simulink model "twoaxis_camera_gantry_Solution_OHackett"  (R2021b)
settings: Solver=ode23t  StartTime=0.0  StopTime=50  MaxStep=0.01  RelTol=1e-3  EnableMultiTasking=on
model workspace: external: MATLAB File gantryParams.m (data not in the file)
values from neighbouring files (symbols this model uses):
  endSupport = struct    [gantryParams.m]
  endSupportZ = struct    [gantryParams.m]
  leadScrew = struct    [gantryParams.m]
  leadScrewZ = struct    [gantryParams.m]
  rail = struct    [gantryParams.m]
  railZ = struct    [gantryParams.m]
  runner = struct    [gantryParams.m]
  runnerZ = struct    [gantryParams.m]
undefined symbols (not defined in the file or in its folder): X, Y, Z
libraries: sm_lib x81, nesl_utility x15, sm_linear_actuator_lib x14, fl_lib x8, ee_lib x3, slpidlib x2, dspsrcs4 x2, mspsensorlib x1
(part 4 of 4)

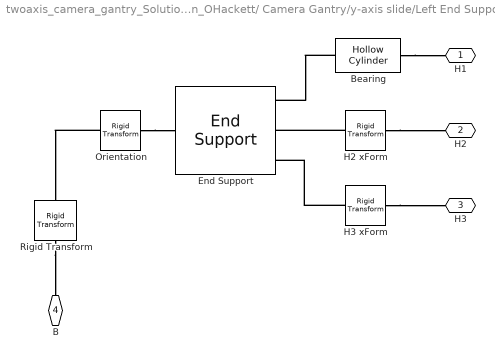
== system twoaxis_camera_gantry_Solution_OHackett/	Camera Gantry/y-axis slide/Left End Support ==
  Bearing : sm_linear_actuator_lib/Hollow Cylinder  StatePerturbationForJacobian=1.0e-05  R=R1+T  T=T  L=D  rho=rho  color=bColor
      settings: SourceProductBaseCode=MS
  End Support : sm_linear_actuator_lib/End Support  StatePerturbationForJacobian=1.0e-05  H=H  W=W  D=D  R1=R1+T  R2=R2  hole1_offset=hole1_offset  hole2_offset=hole2_offset  hole3_offset=hole3_offset  rho=rho  color=sColor
      settings: SourceProductBaseCode=MS
  H2 xForm : sm_lib/Frames and Transforms/Rigid Transform  StatePerturbationForJacobian=1.0e-05  TranslationMethod=StandardAxis  TranslationStandardOffset=D/2  TranslationLengthUnit=mm  TranslationStandardAxis=-Z  TranslationCartesianOffset=[0 0 0]  TranslationROffset=0  TranslationROffsetUnits=m  TranslationZOffset=0  TranslationZOffsetUnits=m  TranslationThetaOffset=0  TranslationThetaOffsetUnits=deg  RotationMethod=None  RotationAngleUnits=deg  RotationStandardAxis=+Z  RotationAngle=0.0  RotationArbitraryAxis=[0 0 1]  FollAlignAxisA=+X  BaseAlignAxisA=+Y  FollAlignAxisB=+Y  BaseAlignAxisB=+Z  RotationSequenceAxes=FollowerAxes  RotationSequence=XYX  RotationSequenceAngles=[0 0 0]  RotationSequenceAnglesUnits=deg  RotationMatrix=[1 0 0; 0 1 0; 0 0 1]
  H3 xForm : sm_lib/Frames and Transforms/Rigid Transform  StatePerturbationForJacobian=1.0e-05  TranslationMethod=StandardAxis  TranslationStandardOffset=D/2  TranslationLengthUnit=mm  TranslationStandardAxis=-Z  TranslationCartesianOffset=[0 0 0]  TranslationROffset=0  TranslationROffsetUnits=m  TranslationZOffset=0  TranslationZOffsetUnits=m  TranslationThetaOffset=0  TranslationThetaOffsetUnits=deg  RotationMethod=None  RotationAngleUnits=deg  RotationStandardAxis=+Z  RotationAngle=0.0  RotationArbitraryAxis=[0 0 1]  FollAlignAxisA=+X  BaseAlignAxisA=+Y  FollAlignAxisB=+Y  BaseAlignAxisB=+Z  RotationSequenceAxes=FollowerAxes  RotationSequence=XYX  RotationSequenceAngles=[0 0 0]  RotationSequenceAnglesUnits=deg  RotationMatrix=[1 0 0; 0 1 0; 0 0 1]
  Orientation : sm_lib/Frames and Transforms/Rigid Transform  StatePerturbationForJacobian=1.0e-05  TranslationMethod=None  TranslationStandardOffset=0  TranslationLengthUnit=m  TranslationStandardAxis=+Z  TranslationCartesianOffset=[0 0 0]  TranslationROffset=0  TranslationROffsetUnits=m  TranslationZOffset=0  TranslationZOffsetUnits=m  TranslationThetaOffset=0  TranslationThetaOffsetUnits=deg  RotationMethod=AlignedAxes  RotationAngleUnits=deg  RotationStandardAxis=+Z  RotationAngle=0.0  RotationArbitraryAxis=[0 0 1]  FollAlignAxisA=+Z  BaseAlignAxisA=+Y  FollAlignAxisB=+Y  BaseAlignAxisB=+Z  RotationSequenceAxes=FollowerAxes  RotationSequence=XYX  RotationSequenceAngles=[0 0 0]  RotationSequenceAnglesUnits=deg  RotationMatrix=[1 0 0; 0 1 0; 0 0 1]
  Rigid Transform : sm_lib/Frames and Transforms/Rigid Transform  TranslationMethod=Cartesian  TranslationStandardOffset=-5  TranslationLengthUnit=mm  TranslationStandardAxis=+Y  TranslationCartesianOffset=[0 -8 25]  TranslationROffset=0  TranslationROffsetUnits=m  TranslationZOffset=0  TranslationZOffsetUnits=m  TranslationThetaOffset=0  TranslationThetaOffsetUnits=deg  RotationMethod=None  RotationAngleUnits=deg  RotationStandardAxis=+Y  RotationAngle=0.0  RotationArbitraryAxis=[0 0 1]  FollAlignAxisA=+X  BaseAlignAxisA=+Y  FollAlignAxisB=+Y  BaseAlignAxisB=+Z  RotationSequenceAxes=FollowerAxes  RotationSequence=XYX  RotationSequenceAngles=[0 0 0]  RotationSequenceAnglesUnits=deg  RotationMatrix=[1 0 0; 0 1 0; 0 0 1]
  H1 : PMIOPort  StatePerturbationForJacobian=1.0e-05  Side=Right
  H2 : PMIOPort  StatePerturbationForJacobian=1.0e-05  Port=2  Side=Right
  H3 : PMIOPort  StatePerturbationForJacobian=1.0e-05  Port=3  Side=Right
  B : PMIOPort  Port=4  Side=Left
  connections:
  Orientation/LConn1 -- Rigid Transform/LConn1
  Bearing/RConn1 -- End Support/RConn1
  H2 xForm/LConn1 -- End Support/RConn2
  H2 xForm/RConn1 -- H2/RConn1
  H3 xForm/RConn1 -- H3/RConn1
  H3 xForm/LConn1 -- End Support/RConn3
  Bearing/LConn1 -- H1/RConn1
  Orientation/RConn1 -- End Support/LConn1
  Rigid Transform/RConn1 -- B/RConn1

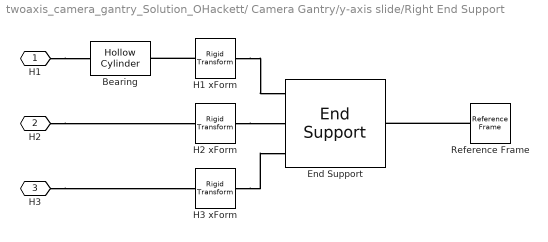
== system twoaxis_camera_gantry_Solution_OHackett/	Camera Gantry/y-axis slide/Right End Support ==
  Bearing : sm_linear_actuator_lib/Hollow Cylinder  StatePerturbationForJacobian=1.0e-05  R=R1+T  T=T  L=D  rho=rho  color=bColor
      settings: SourceProductBaseCode=MS
  End Support : sm_linear_actuator_lib/End Support  StatePerturbationForJacobian=1.0e-05  H=H  W=W  D=D  R1=R1+T  R2=R2  hole1_offset=hole1_offset  hole2_offset=hole2_offset  hole3_offset=hole3_offset  rho=rho  color=sColor
      settings: SourceProductBaseCode=MS
  H1 xForm : sm_lib/Frames and Transforms/Rigid Transform  StatePerturbationForJacobian=1.0e-05  TranslationMethod=None  TranslationStandardOffset=0  TranslationLengthUnit=m  TranslationStandardAxis=+Z  TranslationCartesianOffset=[0 0 0]  TranslationROffset=0  TranslationROffsetUnits=m  TranslationZOffset=0  TranslationZOffsetUnits=m  TranslationThetaOffset=0  TranslationThetaOffsetUnits=deg  RotationMethod=AlignedAxes  RotationAngleUnits=deg  RotationStandardAxis=+Z  RotationAngle=0.0  RotationArbitraryAxis=[0 0 1]  FollAlignAxisA=+Z  BaseAlignAxisA=-Z  FollAlignAxisB=+Y  BaseAlignAxisB=+Y  RotationSequenceAxes=FollowerAxes  RotationSequence=XYX  RotationSequenceAngles=[0 0 0]  RotationSequenceAnglesUnits=deg  RotationMatrix=[1 0 0; 0 1 0; 0 0 1]
  H2 xForm : sm_lib/Frames and Transforms/Rigid Transform  StatePerturbationForJacobian=1.0e-05  TranslationMethod=StandardAxis  TranslationStandardOffset=D/2  TranslationLengthUnit=mm  TranslationStandardAxis=+Z  TranslationCartesianOffset=[0 0 0]  TranslationROffset=0  TranslationROffsetUnits=m  TranslationZOffset=0  TranslationZOffsetUnits=m  TranslationThetaOffset=0  TranslationThetaOffsetUnits=deg  RotationMethod=AlignedAxes  RotationAngleUnits=deg  RotationStandardAxis=+Z  RotationAngle=0.0  RotationArbitraryAxis=[0 0 1]  FollAlignAxisA=+Z  BaseAlignAxisA=-Z  FollAlignAxisB=+Y  BaseAlignAxisB=+Y  RotationSequenceAxes=FollowerAxes  RotationSequence=XYX  RotationSequenceAngles=[0 0 0]  RotationSequenceAnglesUnits=deg  RotationMatrix=[1 0 0; 0 1 0; 0 0 1]
  H3 xForm : sm_lib/Frames and Transforms/Rigid Transform  StatePerturbationForJacobian=1.0e-05  TranslationMethod=StandardAxis  TranslationStandardOffset=D/2  TranslationLengthUnit=mm  TranslationStandardAxis=+Z  TranslationCartesianOffset=[0 0 0]  TranslationROffset=0  TranslationROffsetUnits=m  TranslationZOffset=0  TranslationZOffsetUnits=m  TranslationThetaOffset=0  TranslationThetaOffsetUnits=deg  RotationMethod=AlignedAxes  RotationAngleUnits=deg  RotationStandardAxis=+Z  RotationAngle=0.0  RotationArbitraryAxis=[0 0 1]  FollAlignAxisA=+Z  BaseAlignAxisA=-Z  FollAlignAxisB=+Y  BaseAlignAxisB=+Y  RotationSequenceAxes=FollowerAxes  RotationSequence=XYX  RotationSequenceAngles=[0 0 0]  RotationSequenceAnglesUnits=deg  RotationMatrix=[1 0 0; 0 1 0; 0 0 1]
  Reference Frame : sm_lib/Frames and Transforms/Reference Frame  StatePerturbationForJacobian=1.0e-05
  H1 : PMIOPort  StatePerturbationForJacobian=1.0e-05  Side=Left
  H2 : PMIOPort  StatePerturbationForJacobian=1.0e-05  Port=2  Side=Left
  H3 : PMIOPort  StatePerturbationForJacobian=1.0e-05  Port=3  Side=Left
  connections:
  H1 xForm/LConn1 -- End Support/RConn1
  H3 xForm/LConn1 -- End Support/RConn3
  H2 xForm/LConn1 -- End Support/RConn2
  H1 xForm/RConn1 -- Bearing/RConn1
  H1/RConn1 -- Bearing/LConn1
  H2/RConn1 -- H2 xForm/RConn1
  H3/RConn1 -- H3 xForm/RConn1
  Reference Frame/RConn1 -- End Support/LConn1

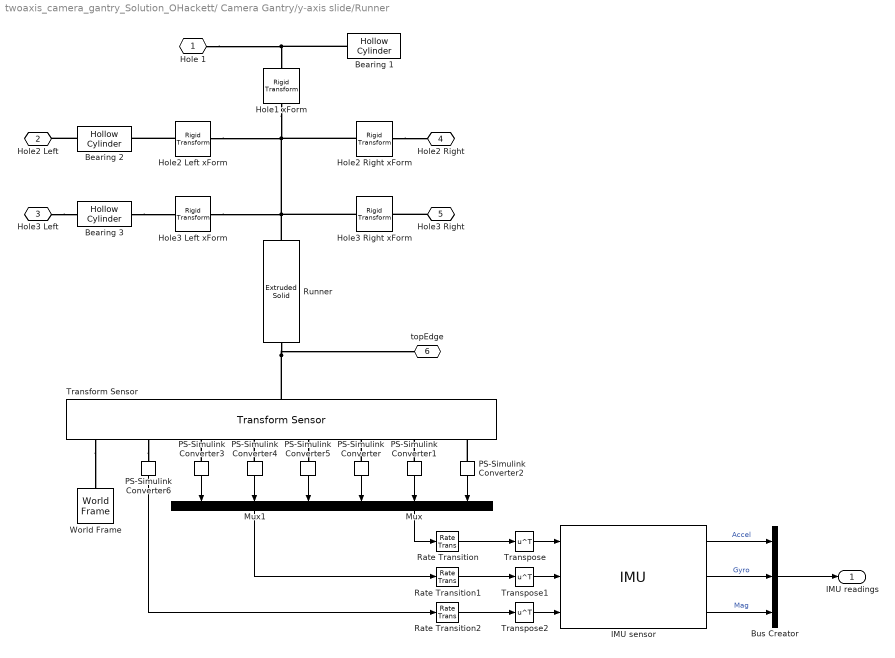
== system twoaxis_camera_gantry_Solution_OHackett/	Camera Gantry/y-axis slide/Runner ==
  Bearing 1 : sm_linear_actuator_lib/Hollow Cylinder  StatePerturbationForJacobian=1.0e-05  R=R1+T  T=T  L=D  rho=rho  color=bColor
      settings: SourceProductBaseCode=MS
  Bearing 2 : sm_linear_actuator_lib/Hollow Cylinder  StatePerturbationForJacobian=1.0e-05  R=R2+T  T=T  L=D  rho=rho  color=bColor
      settings: SourceProductBaseCode=MS
  Bearing 3 : sm_linear_actuator_lib/Hollow Cylinder  StatePerturbationForJacobian=1.0e-05  R=R2+T  T=T  L=D  rho=rho  color=bColor
      settings: SourceProductBaseCode=MS
  Bus Creator : BusCreator  Inputs=3
  Hole1 xForm : sm_lib/Frames and Transforms/Rigid Transform  StatePerturbationForJacobian=1.0e-05  TranslationMethod=Cartesian  TranslationStandardOffset=0  TranslationLengthUnit=mm  TranslationStandardAxis=+Z  TranslationCartesianOffset=[hole1_offset 0]  TranslationROffset=0  TranslationROffsetUnits=m  TranslationZOffset=0  TranslationZOffsetUnits=m  TranslationThetaOffset=0  TranslationThetaOffsetUnits=deg  RotationMethod=None  RotationAngleUnits=deg  RotationStandardAxis=+Z  RotationAngle=0.0  RotationArbitraryAxis=[0 0 1]  FollAlignAxisA=+X  BaseAlignAxisA=+Y  FollAlignAxisB=+Y  BaseAlignAxisB=+Z  RotationSequenceAxes=FollowerAxes  RotationSequence=XYX  RotationSequenceAngles=[0 0 0]  RotationSequenceAnglesUnits=deg  RotationMatrix=[1 0 0; 0 1 0; 0 0 1]
  Hole2 Left xForm : sm_lib/Frames and Transforms/Rigid Transform  StatePerturbationForJacobian=1.0e-05  TranslationMethod=Cartesian  TranslationStandardOffset=0  TranslationLengthUnit=mm  TranslationStandardAxis=+Z  TranslationCartesianOffset=[hole2_offset 0]  TranslationROffset=0  TranslationROffsetUnits=m  TranslationZOffset=0  TranslationZOffsetUnits=m  TranslationThetaOffset=0  TranslationThetaOffsetUnits=deg  RotationMethod=None  RotationAngleUnits=deg  RotationStandardAxis=+Z  RotationAngle=0.0  RotationArbitraryAxis=[0 0 1]  FollAlignAxisA=+X  BaseAlignAxisA=+Y  FollAlignAxisB=+Y  BaseAlignAxisB=+Z  RotationSequenceAxes=FollowerAxes  RotationSequence=XYX  RotationSequenceAngles=[0 0 0]  RotationSequenceAnglesUnits=deg  RotationMatrix=[1 0 0; 0 1 0; 0 0 1]
  Hole2 Right xForm : sm_lib/Frames and Transforms/Rigid Transform  StatePerturbationForJacobian=1.0e-05  TranslationMethod=Cartesian  TranslationStandardOffset=0  TranslationLengthUnit=mm  TranslationStandardAxis=+Z  TranslationCartesianOffset=[hole2_offset D/2]  TranslationROffset=0  TranslationROffsetUnits=m  TranslationZOffset=0  TranslationZOffsetUnits=m  TranslationThetaOffset=0  TranslationThetaOffsetUnits=deg  RotationMethod=AlignedAxes  RotationAngleUnits=deg  RotationStandardAxis=+Z  RotationAngle=0.0  RotationArbitraryAxis=[0 0 1]  FollAlignAxisA=+Z  BaseAlignAxisA=-Z  FollAlignAxisB=+Y  BaseAlignAxisB=+Y  RotationSequenceAxes=FollowerAxes  RotationSequence=XYX  RotationSequenceAngles=[0 0 0]  RotationSequenceAnglesUnits=deg  RotationMatrix=[1 0 0; 0 1 0; 0 0 1]
  Hole3 Left xForm : sm_lib/Frames and Transforms/Rigid Transform  StatePerturbationForJacobian=1.0e-05  TranslationMethod=Cartesian  TranslationStandardOffset=0  TranslationLengthUnit=mm  TranslationStandardAxis=+Z  TranslationCartesianOffset=[hole3_offset 0]  TranslationROffset=0  TranslationROffsetUnits=m  TranslationZOffset=0  TranslationZOffsetUnits=m  TranslationThetaOffset=0  TranslationThetaOffsetUnits=deg  RotationMethod=None  RotationAngleUnits=deg  RotationStandardAxis=+Z  RotationAngle=0.0  RotationArbitraryAxis=[0 0 1]  FollAlignAxisA=+X  BaseAlignAxisA=+Y  FollAlignAxisB=+Y  BaseAlignAxisB=+Z  RotationSequenceAxes=FollowerAxes  RotationSequence=XYX  RotationSequenceAngles=[0 0 0]  RotationSequenceAnglesUnits=deg  RotationMatrix=[1 0 0; 0 1 0; 0 0 1]
  Hole3 Right xForm : sm_lib/Frames and Transforms/Rigid Transform  StatePerturbationForJacobian=1.0e-05  TranslationMethod=Cartesian  TranslationStandardOffset=0  TranslationLengthUnit=mm  TranslationStandardAxis=+Z  TranslationCartesianOffset=[hole3_offset D/2]  TranslationROffset=0  TranslationROffsetUnits=m  TranslationZOffset=0  TranslationZOffsetUnits=m  TranslationThetaOffset=0  TranslationThetaOffsetUnits=deg  RotationMethod=AlignedAxes  RotationAngleUnits=deg  RotationStandardAxis=+Z  RotationAngle=0.0  RotationArbitraryAxis=[0 0 1]  FollAlignAxisA=+Z  BaseAlignAxisA=-Z  FollAlignAxisB=+Y  BaseAlignAxisB=+Y  RotationSequenceAxes=FollowerAxes  RotationSequence=XYX  RotationSequenceAngles=[0 0 0]  RotationSequenceAnglesUnits=deg  RotationMatrix=[1 0 0; 0 1 0; 0 0 1]
  IMU sensor : mspsensorlib/IMU  DispRefFrame=ENU  Temperature=25  MagneticFieldNED=[ 27.5550, -2.4169, -16.0849 ]  MagneticFieldENU=[ -2.4169, 27.5550, 16.0849 ]  SeedDouble=67  SimulateUsing=Code generation  AccelParamsMeasurementRange=Inf  AccelParamsResolution=0  AccelParamsConstantBias=[ 0, 0, 0 ]  AccelParamsAxesMisalignment=[ 100, 0, 0; 0, 100, 0; 0, 0, 100 ]  AccelParamsNoiseDensity=[ 0, 0, 0 ]  AccelParamsBiasInstability=[ 0, 0, 0 ]  AccelParamsRandomWalk=[ 0, 0, 0 ]  AccelParamsTemperatureBias=[ 0, 0, 0 ]  AccelParamsTemperatureScaleFactor=[ 0, 0, 0 ]  GyroParamsMeasurementRange=Inf  GyroParamsResolution=0  GyroParamsConstantBias=[ 0, 0, 0 ]  GyroParamsAxesMisalignment=[ 100, 0, 0; 0, 100, 0; 0, 0, 100 ]  GyroParamsAccelerationBias=[ 0, 0, 0 ]  GyroParamsNoiseDensity=[ 0, 0, 0 ]  GyroParamsBiasInstability=[ 0, 0, 0 ]  GyroParamsRandomWalk=[ 0, 0, 0 ]  GyroParamsTemperatureBias=[ 0, 0, 0 ]  GyroParamsTemperatureScaleFactor=[ 0, 0, 0 ]  MagParamsMeasurementRange=Inf  MagParamsResolution=0  MagParamsConstantBias=[ 0, 0, 0 ]  MagParamsAxesMisalignment=[ 100, 0, 0; 0, 100, 0; 0, 0, 100 ]  MagParamsNoiseDensity=[ 0, 0, 0 ]  MagParamsBiasInstability=[ 0, 0, 0 ]  MagParamsRandomWalk=[ 0, 0, 0 ]  MagParamsTemperatureBias=[ 0, 0, 0 ]  MagParamsTemperatureScaleFactor=[ 0, 0, 0 ]
      settings: SourceProductBaseCode=TF,NV
  Mux : Mux  Inputs=3
  Mux1 : Mux  Inputs=3
  PS-Simulink Converter{,1..6} (7 alike) : nesl_utility/PS-Simulink Converter  PhysicalDomain=network_engine_domain  SubClassName=ps_output  LeftPortType=input  RightPortType=output  PseudoPeriodic=off  Frequencies=[]  Unit=inherit  AffineConversion=off
      settings: SourceProductBaseCode=PW,SS
  Rate Transition : RateTransition  OutPortSampleTime=1e-2
  Rate Transition1 : RateTransition  OutPortSampleTime=1e-2
  Rate Transition2 : RateTransition  OutPortSampleTime=1e-2
  Runner : sm_lib/Body Elements/Extruded Solid  StatePerturbationForJacobian=1.0e-05  GraphicAmbientColor=[0.15 0.15 0.15 1.0]  BasedOnType=Density  CenterOfMass=[0 0 0]  CenterOfMassUnits=m  GraphicDiffuseColor=rColor  ExportConvexHullGeometry=off  ExtrusionCrossSection=extrusion_points  ExtrusionCrossSectionUnits=mm  Density=rho  DensityUnits=kg/(m^3)  DoExposeReferenceFrame=on  GraphicEmissiveColor=[0.0 0.0 0.0 1.0]  ExportEntireGeometry=off  ExtrusionLength=D  ExtrusionLengthUnits=mm  ExtrusionType=General  SerializedFrames=<Frames><Frame><Id>Frame1</Id><Value><Name>topEdge</Name><Origin><Source>GeometricFeature</Source><FeatureName>side curve 46</FeatureName></Origin><PrimaryAxis><DefinedDirection>+Z</DefinedDirection><Source>ReferenceFrame</Source><SourceDirection>+Z</SourceDirection><FeatureName></FeatureName></PrimaryAxis><SecondaryAxis><DefinedDirection>+X</DefinedDirection><Source>ReferenceFrame</Source><SourceDirection>+X</SourceDirection><FeatureName></FeatureName></SecondaryAxis></Value></Frame></Frames>  MarkerShape=Sphere  MarkerSize=10  GraphicType=FromGeometry  InertiaType=CalculateFromGeometry  Mass=1  MassUnits=kg  MomentsOfInertia=[1 1 1]  MomentsOfInertiaUnits=kg*m^2  PolygonNumSides=3  GraphicOpacity=0.9  PolygonOuterRadius=1  PolygonOuterRadiusUnits=m  ProductsOfInertia=[0 0 0]  ProductsOfInertiaUnits=kg*m^2  GraphicShininess=75  GraphicSpecularColor=[0.5 0.5 0.5 1.0]  GraphicVisPropType=SimpleVisualProperties
  Transform Sensor : sm_lib/Frames and Transforms/Transform Sensor  MeasurementFrame=World  SenseAngle=off  SenseAxis=off  SenseAngle1=off  SenseAngle2=off  SenseAngle3=off  SenseQ=on  SenseR=off  SenseOmegaX=on  SenseOmegaY=on  SenseOmegaZ=on  SenseOmega1=off  SenseOmega2=off  SenseOmega3=off  SenseQDot=off  SenseRDot=off  SenseAlphaX=off  SenseAlphaY=off  SenseAlphaZ=off  SenseAlpha1=off  SenseAlpha2=off  SenseAlpha3=off  SenseQDDot=off  SenseRDDot=off  SenseX=off  SenseY=off  SenseZ=off  SenseRad=off  SenseAzim=off  SenseDist=off  SenseInc=off  SenseXDot=off  SenseYDot=off  SenseZDot=off  SenseRadDot=off  SenseAzimDot=off  SenseDistDot=off  SenseIncDot=off  SenseXDDot=on  SenseYDDot=on  SenseZDDot=on  SenseRadDDot=off  SenseAzimDDot=off  SenseDistDDot=off  SenseIncDDot=off
  Transpose : Math  Operator=transpose  SaturateOnIntegerOverflow=on
  Transpose1 : Math  Operator=transpose  SaturateOnIntegerOverflow=on
  Transpose2 : Math  Operator=transpose  SaturateOnIntegerOverflow=on
  World Frame : sm_lib/Frames and Transforms/World Frame
  Hole 1 : PMIOPort  StatePerturbationForJacobian=1.0e-05  Side=Left
  Hole2 Left : PMIOPort  StatePerturbationForJacobian=1.0e-05  Port=2  Side=Left
  Hole3 Left : PMIOPort  StatePerturbationForJacobian=1.0e-05  Port=3  Side=Left
  Hole2 Right : PMIOPort  StatePerturbationForJacobian=1.0e-05  Port=4  Side=Right
  Hole3 Right : PMIOPort  StatePerturbationForJacobian=1.0e-05  Port=5  Side=Right
  topEdge : PMIOPort  Port=6  Side=Right
  IMU readings : Outport
  wires:
  PS-Simulink Converter/1 -> Mux/1
  PS-Simulink Converter1/1 -> Mux/2
  PS-Simulink Converter2/1 -> Mux/3
  Mux/1 -> Rate Transition/1
  PS-Simulink Converter5/1 -> Mux1/3
  PS-Simulink Converter4/1 -> Mux1/2
  PS-Simulink Converter3/1 -> Mux1/1
  Mux1/1 -> Rate Transition1/1
  IMU sensor/1 -> Bus Creator/1  "Accel"
  IMU sensor/2 -> Bus Creator/2  "Gyro"
  IMU sensor/3 -> Bus Creator/3  "Mag"
  Bus Creator/1 -> IMU readings/1
  Transpose/1 -> IMU sensor/1
  Transpose1/1 -> IMU sensor/2
  PS-Simulink Converter6/1 -> Rate Transition2/1
  Transpose2/1 -> IMU sensor/3
  Rate Transition/1 -> Transpose/1
  Rate Transition1/1 -> Transpose1/1
  Rate Transition2/1 -> Transpose2/1
  connections:
  Hole2 Left xForm/RConn1 -- Bearing 2/RConn1
  Bearing 3/RConn1 -- Hole3 Left xForm/RConn1
  Hole2 Right xForm/RConn1 -- Hole2 Right/RConn1
  Hole3 Left/RConn1 -- Bearing 3/LConn1
  Hole3 Right/RConn1 -- Hole3 Right xForm/RConn1
  Bearing 2/LConn1 -- Hole2 Left/RConn1
  Bearing 1/RConn1 -- Hole1 xForm/RConn1 -- Hole 1/RConn1
  Hole3 Left xForm/LConn1 -- Hole3 Right xForm/LConn1 -- Hole1 xForm/LConn1 -- Hole2 Left xForm/LConn1 -- Hole2 Right xForm/LConn1 -- Runner/RConn1
  Runner/LConn1 -- topEdge/RConn1 -- Transform Sensor/LConn1
  Transform Sensor/RConn1 -- World Frame/RConn1
  PS-Simulink Converter/LConn1 -- Transform Sensor/RConn6
  PS-Simulink Converter1/LConn1 -- Transform Sensor/RConn7
  PS-Simulink Converter2/LConn1 -- Transform Sensor/RConn8
  Transform Sensor/RConn5 -- PS-Simulink Converter5/LConn1
  PS-Simulink Converter4/LConn1 -- Transform Sensor/RConn4
  PS-Simulink Converter3/LConn1 -- Transform Sensor/RConn3
  Transform Sensor/RConn2 -- PS-Simulink Converter6/LConn1

== system twoaxis_camera_gantry_Solution_OHackett/	Camera Gantry/z-axis slide/Guide Rail1 ==
  Left xForm : sm_lib/Frames and Transforms/Rigid Transform  StatePerturbationForJacobian=1.0e-05  TranslationMethod=StandardAxis  TranslationStandardOffset=L/2  TranslationLengthUnit=mm  TranslationStandardAxis=+Z  TranslationCartesianOffset=[0 0 0]  TranslationROffset=0  TranslationROffsetUnits=m  TranslationZOffset=0  TranslationZOffsetUnits=m  TranslationThetaOffset=0  TranslationThetaOffsetUnits=deg  RotationMethod=AlignedAxes  RotationAngleUnits=deg  RotationStandardAxis=+Z  RotationAngle=0.0  RotationArbitraryAxis=[0 0 1]  FollAlignAxisA=+Z  BaseAlignAxisA=-Z  FollAlignAxisB=+Y  BaseAlignAxisB=+Y  RotationSequenceAxes=FollowerAxes  RotationSequence=XYX  RotationSequenceAngles=[0 0 0]  RotationSequenceAnglesUnits=deg  RotationMatrix=[1 0 0; 0 1 0; 0 0 1]
  Rail : sm_lib/Body Elements/Cylindrical Solid  StatePerturbationForJacobian=1.0e-05  GraphicAmbientColor=[0.15 0.15 0.15 1.0]  BasedOnType=Density  CenterOfMass=[0 0 0]  CenterOfMassUnits=m  GraphicDiffuseColor=color  CylinderLength=L  CylinderLengthUnits=mm  CylinderRadius=R  CylinderRadiusUnits=mm  Density=rho  DensityUnits=kg/(m^3)  DoExposeReferenceFrame=on  GraphicEmissiveColor=[0.0 0.0 0.0 1.0]  ExportEntireGeometry=off  SerializedFrames=<Frames/>  MarkerShape=Sphere  MarkerSize=10  GraphicType=FromGeometry  InertiaType=CalculateFromGeometry  Mass=1  MassUnits=kg  MomentsOfInertia=[1 1 1]  MomentsOfInertiaUnits=kg*m^2  GraphicOpacity=1.0  ProductsOfInertia=[0 0 0]  ProductsOfInertiaUnits=kg*m^2  GraphicShininess=75  GraphicSpecularColor=[0.5 0.5 0.5 1.0]  GraphicVisPropType=SimpleVisualProperties
  Right xForm : sm_lib/Frames and Transforms/Rigid Transform  StatePerturbationForJacobian=1.0e-05  TranslationMethod=StandardAxis  TranslationStandardOffset=L/2  TranslationLengthUnit=mm  TranslationStandardAxis=-Z  TranslationCartesianOffset=[0 0 0]  TranslationROffset=0  TranslationROffsetUnits=m  TranslationZOffset=0  TranslationZOffsetUnits=m  TranslationThetaOffset=0  TranslationThetaOffsetUnits=deg  RotationMethod=None  RotationAngleUnits=deg  RotationStandardAxis=+Z  RotationAngle=0.0  RotationArbitraryAxis=[0 0 1]  FollAlignAxisA=+Z  BaseAlignAxisA=+Z  FollAlignAxisB=+Y  BaseAlignAxisB=+Y  RotationSequenceAxes=FollowerAxes  RotationSequence=XYX  RotationSequenceAngles=[0 0 0]  RotationSequenceAnglesUnits=deg  RotationMatrix=[1 0 0; 0 1 0; 0 0 1]
  L : PMIOPort  StatePerturbationForJacobian=1.0e-05  Side=Left
  R : PMIOPort  StatePerturbationForJacobian=1.0e-05  Port=2  Side=Right
  connections:
  Right xForm/LConn1 -- Rail/RConn1 -- Left xForm/LConn1
  Right xForm/RConn1 -- R/RConn1
  Left xForm/RConn1 -- L/RConn1

== system twoaxis_camera_gantry_Solution_OHackett/	Camera Gantry/z-axis slide/Guide Rail2 ==
  Left xForm : sm_lib/Frames and Transforms/Rigid Transform  StatePerturbationForJacobian=1.0e-05  TranslationMethod=StandardAxis  TranslationStandardOffset=L/2  TranslationLengthUnit=mm  TranslationStandardAxis=+Z  TranslationCartesianOffset=[0 0 0]  TranslationROffset=0  TranslationROffsetUnits=m  TranslationZOffset=0  TranslationZOffsetUnits=m  TranslationThetaOffset=0  TranslationThetaOffsetUnits=deg  RotationMethod=AlignedAxes  RotationAngleUnits=deg  RotationStandardAxis=+Z  RotationAngle=0.0  RotationArbitraryAxis=[0 0 1]  FollAlignAxisA=+Z  BaseAlignAxisA=-Z  FollAlignAxisB=+Y  BaseAlignAxisB=+Y  RotationSequenceAxes=FollowerAxes  RotationSequence=XYX  RotationSequenceAngles=[0 0 0]  RotationSequenceAnglesUnits=deg  RotationMatrix=[1 0 0; 0 1 0; 0 0 1]
  Rail : sm_lib/Body Elements/Cylindrical Solid  StatePerturbationForJacobian=1.0e-05  GraphicAmbientColor=[0.15 0.15 0.15 1.0]  BasedOnType=Density  CenterOfMass=[0 0 0]  CenterOfMassUnits=m  GraphicDiffuseColor=color  CylinderLength=L  CylinderLengthUnits=mm  CylinderRadius=R  CylinderRadiusUnits=mm  Density=rho  DensityUnits=kg/(m^3)  DoExposeReferenceFrame=on  GraphicEmissiveColor=[0.0 0.0 0.0 1.0]  ExportEntireGeometry=off  SerializedFrames=<Frames/>  MarkerShape=Sphere  MarkerSize=10  GraphicType=FromGeometry  InertiaType=CalculateFromGeometry  Mass=1  MassUnits=kg  MomentsOfInertia=[1 1 1]  MomentsOfInertiaUnits=kg*m^2  GraphicOpacity=1.0  ProductsOfInertia=[0 0 0]  ProductsOfInertiaUnits=kg*m^2  GraphicShininess=75  GraphicSpecularColor=[0.5 0.5 0.5 1.0]  GraphicVisPropType=SimpleVisualProperties
  Right xForm : sm_lib/Frames and Transforms/Rigid Transform  StatePerturbationForJacobian=1.0e-05  TranslationMethod=StandardAxis  TranslationStandardOffset=L/2  TranslationLengthUnit=mm  TranslationStandardAxis=-Z  TranslationCartesianOffset=[0 0 0]  TranslationROffset=0  TranslationROffsetUnits=m  TranslationZOffset=0  TranslationZOffsetUnits=m  TranslationThetaOffset=0  TranslationThetaOffsetUnits=deg  RotationMethod=None  RotationAngleUnits=deg  RotationStandardAxis=+Z  RotationAngle=0.0  RotationArbitraryAxis=[0 0 1]  FollAlignAxisA=+Z  BaseAlignAxisA=+Z  FollAlignAxisB=+Y  BaseAlignAxisB=+Y  RotationSequenceAxes=FollowerAxes  RotationSequence=XYX  RotationSequenceAngles=[0 0 0]  RotationSequenceAnglesUnits=deg  RotationMatrix=[1 0 0; 0 1 0; 0 0 1]
  L : PMIOPort  StatePerturbationForJacobian=1.0e-05  Side=Left
  R : PMIOPort  StatePerturbationForJacobian=1.0e-05  Port=2  Side=Right
  connections:
  Right xForm/LConn1 -- Rail/RConn1 -- Left xForm/LConn1
  Right xForm/RConn1 -- R/RConn1
  Left xForm/RConn1 -- L/RConn1

== system twoaxis_camera_gantry_Solution_OHackett/	Camera Gantry/z-axis slide/Lead Screw ==
  Left : sm_lib/Body Elements/Extruded Solid  StatePerturbationForJacobian=1.0e-05  GraphicAmbientColor=[0.15 0.15 0.15 1.0]  BasedOnType=Density  CenterOfMass=[0 0 0]  CenterOfMassUnits=m  GraphicDiffuseColor=oColor  ExportConvexHullGeometry=off  ExtrusionCrossSection=left_section  ExtrusionCrossSectionUnits=mm  Density=rho  DensityUnits=kg/(m^3)  DoExposeReferenceFrame=on  GraphicEmissiveColor=[0.0 0.0 0.0 1.0]  ExportEntireGeometry=off  ExtrusionLength=L  ExtrusionLengthUnits=mm  ExtrusionType=General  SerializedFrames=<Frames/>  MarkerShape=Sphere  MarkerSize=10  GraphicType=FromGeometry  InertiaType=CalculateFromGeometry  Mass=1  MassUnits=kg  MomentsOfInertia=[1 1 1]  MomentsOfInertiaUnits=kg*m^2  PolygonNumSides=3  GraphicOpacity=1.0  PolygonOuterRadius=1  PolygonOuterRadiusUnits=m  ProductsOfInertia=[0 0 0]  ProductsOfInertiaUnits=kg*m^2  GraphicShininess=75  GraphicSpecularColor=[0.5 0.5 0.5 1.0]  GraphicVisPropType=SimpleVisualProperties
  Left xForm : sm_lib/Frames and Transforms/Rigid Transform  StatePerturbationForJacobian=1.0e-05  TranslationMethod=StandardAxis  TranslationStandardOffset=L/2  TranslationLengthUnit=mm  TranslationStandardAxis=+Z  TranslationCartesianOffset=[0 0 0]  TranslationROffset=0  TranslationROffsetUnits=m  TranslationZOffset=0  TranslationZOffsetUnits=m  TranslationThetaOffset=0  TranslationThetaOffsetUnits=deg  RotationMethod=AlignedAxes  RotationAngleUnits=deg  RotationStandardAxis=+Z  RotationAngle=0.0  RotationArbitraryAxis=[0 0 1]  FollAlignAxisA=+Z  BaseAlignAxisA=-Z  FollAlignAxisB=+Y  BaseAlignAxisB=+Y  RotationSequenceAxes=FollowerAxes  RotationSequence=XYX  RotationSequenceAngles=[0 0 0]  RotationSequenceAnglesUnits=deg  RotationMatrix=[1 0 0; 0 1 0; 0 0 1]
  Middle : sm_lib/Body Elements/Extruded Solid  StatePerturbationForJacobian=1.0e-05  GraphicAmbientColor=[0.15 0.15 0.15 1.0]  BasedOnType=Density  CenterOfMass=[0 0 0]  CenterOfMassUnits=m  GraphicDiffuseColor=iColor  ExportConvexHullGeometry=off  ExtrusionCrossSection=middle_section  ExtrusionCrossSectionUnits=mm  Density=rho  DensityUnits=kg/(m^3)  DoExposeReferenceFrame=on  GraphicEmissiveColor=[0.0 0.0 0.0 1.0]  ExportEntireGeometry=off  ExtrusionLength=L  ExtrusionLengthUnits=mm  ExtrusionType=General  SerializedFrames=<Frames/>  MarkerShape=Sphere  MarkerSize=10  GraphicType=FromGeometry  InertiaType=CalculateFromGeometry  Mass=1  MassUnits=kg  MomentsOfInertia=[1 1 1]  MomentsOfInertiaUnits=kg*m^2  PolygonNumSides=3  GraphicOpacity=1.0  PolygonOuterRadius=1  PolygonOuterRadiusUnits=m  ProductsOfInertia=[0 0 0]  ProductsOfInertiaUnits=kg*m^2  GraphicShininess=75  GraphicSpecularColor=[0.5 0.5 0.5 1.0]  GraphicVisPropType=SimpleVisualProperties
  Right : sm_lib/Body Elements/Extruded Solid  StatePerturbationForJacobian=1.0e-05  GraphicAmbientColor=[0.15 0.15 0.15 1.0]  BasedOnType=Density  CenterOfMass=[0 0 0]  CenterOfMassUnits=m  GraphicDiffuseColor=oColor  ExportConvexHullGeometry=off  ExtrusionCrossSection=right_section  ExtrusionCrossSectionUnits=mm  Density=rho  DensityUnits=kg/(m^3)  DoExposeReferenceFrame=on  GraphicEmissiveColor=[0.0 0.0 0.0 1.0]  ExportEntireGeometry=off  ExtrusionLength=L  ExtrusionLengthUnits=mm  ExtrusionType=General  SerializedFrames=<Frames/>  MarkerShape=Sphere  MarkerSize=10  GraphicType=FromGeometry  InertiaType=CalculateFromGeometry  Mass=1  MassUnits=kg  MomentsOfInertia=[1 1 1]  MomentsOfInertiaUnits=kg*m^2  PolygonNumSides=3  GraphicOpacity=1.0  PolygonOuterRadius=1  PolygonOuterRadiusUnits=m  ProductsOfInertia=[0 0 0]  ProductsOfInertiaUnits=kg*m^2  GraphicShininess=75  GraphicSpecularColor=[0.5 0.5 0.5 1.0]  GraphicVisPropType=SimpleVisualProperties
  Right xForm : sm_lib/Frames and Transforms/Rigid Transform  StatePerturbationForJacobian=1.0e-05  TranslationMethod=StandardAxis  TranslationStandardOffset=L/2  TranslationLengthUnit=mm  TranslationStandardAxis=-Z  TranslationCartesianOffset=[0 0 0]  TranslationROffset=0  TranslationROffsetUnits=m  TranslationZOffset=0  TranslationZOffsetUnits=m  TranslationThetaOffset=0  TranslationThetaOffsetUnits=deg  RotationMethod=None  RotationAngleUnits=deg  RotationStandardAxis=+Z  RotationAngle=0.0  RotationArbitraryAxis=[0 0 1]  FollAlignAxisA=+Z  BaseAlignAxisA=+Z  FollAlignAxisB=+Y  BaseAlignAxisB=+Y  RotationSequenceAxes=FollowerAxes  RotationSequence=XYX  RotationSequenceAngles=[0 0 0]  RotationSequenceAnglesUnits=deg  RotationMatrix=[1 0 0; 0 1 0; 0 0 1]
  L : PMIOPort  StatePerturbationForJacobian=1.0e-05  Side=Left
  R : PMIOPort  StatePerturbationForJacobian=1.0e-05  Port=2  Side=Right
  connections:
  Left xForm/RConn1 -- L/RConn1
  Right xForm/RConn1 -- R/RConn1
  Left xForm/LConn1 -- Middle/RConn1 -- Left/RConn1 -- Right/RConn1 -- Right xForm/LConn1

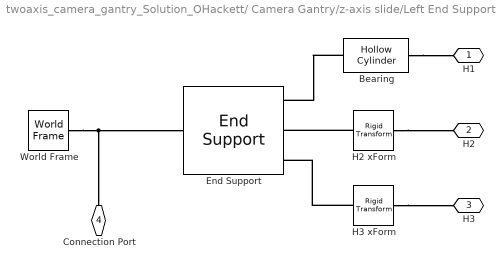
== system twoaxis_camera_gantry_Solution_OHackett/	Camera Gantry/z-axis slide/Left End Support ==
  Bearing : sm_linear_actuator_lib/Hollow Cylinder  StatePerturbationForJacobian=1.0e-05  R=R1+T  T=T  L=D  rho=rho  color=bColor
      settings: SourceProductBaseCode=MS
  End Support : sm_linear_actuator_lib/End Support  StatePerturbationForJacobian=1.0e-05  H=H  W=W  D=D  R1=R1+T  R2=R2  hole1_offset=hole1_offset  hole2_offset=hole2_offset  hole3_offset=hole3_offset  rho=rho  color=sColor
      settings: SourceProductBaseCode=MS
  H2 xForm : sm_lib/Frames and Transforms/Rigid Transform  StatePerturbationForJacobian=1.0e-05  TranslationMethod=StandardAxis  TranslationStandardOffset=D/2  TranslationLengthUnit=mm  TranslationStandardAxis=-Z  TranslationCartesianOffset=[0 0 0]  TranslationROffset=0  TranslationROffsetUnits=m  TranslationZOffset=0  TranslationZOffsetUnits=m  TranslationThetaOffset=0  TranslationThetaOffsetUnits=deg  RotationMethod=None  RotationAngleUnits=deg  RotationStandardAxis=+Z  RotationAngle=0.0  RotationArbitraryAxis=[0 0 1]  FollAlignAxisA=+X  BaseAlignAxisA=+Y  FollAlignAxisB=+Y  BaseAlignAxisB=+Z  RotationSequenceAxes=FollowerAxes  RotationSequence=XYX  RotationSequenceAngles=[0 0 0]  RotationSequenceAnglesUnits=deg  RotationMatrix=[1 0 0; 0 1 0; 0 0 1]
  H3 xForm : sm_lib/Frames and Transforms/Rigid Transform  StatePerturbationForJacobian=1.0e-05  TranslationMethod=StandardAxis  TranslationStandardOffset=D/2  TranslationLengthUnit=mm  TranslationStandardAxis=-Z  TranslationCartesianOffset=[0 0 0]  TranslationROffset=0  TranslationROffsetUnits=m  TranslationZOffset=0  TranslationZOffsetUnits=m  TranslationThetaOffset=0  TranslationThetaOffsetUnits=deg  RotationMethod=None  RotationAngleUnits=deg  RotationStandardAxis=+Z  RotationAngle=0.0  RotationArbitraryAxis=[0 0 1]  FollAlignAxisA=+X  BaseAlignAxisA=+Y  FollAlignAxisB=+Y  BaseAlignAxisB=+Z  RotationSequenceAxes=FollowerAxes  RotationSequence=XYX  RotationSequenceAngles=[0 0 0]  RotationSequenceAnglesUnits=deg  RotationMatrix=[1 0 0; 0 1 0; 0 0 1]
  World Frame : sm_lib/Frames and Transforms/World Frame  StatePerturbationForJacobian=1.0e-05
  H1 : PMIOPort  StatePerturbationForJacobian=1.0e-05  Side=Right
  H2 : PMIOPort  StatePerturbationForJacobian=1.0e-05  Port=2  Side=Right
  H3 : PMIOPort  StatePerturbationForJacobian=1.0e-05  Port=3  Side=Right
  Connection Port : PMIOPort  Port=4  Side=Left
  connections:
  Bearing/LConn1 -- H1/RConn1
  H3 xForm/LConn1 -- End Support/RConn3
  H3 xForm/RConn1 -- H3/RConn1
  H2 xForm/RConn1 -- H2/RConn1
  H2 xForm/LConn1 -- End Support/RConn2
  Bearing/RConn1 -- End Support/RConn1
  World Frame/RConn1 -- End Support/LConn1 -- Connection Port/RConn1

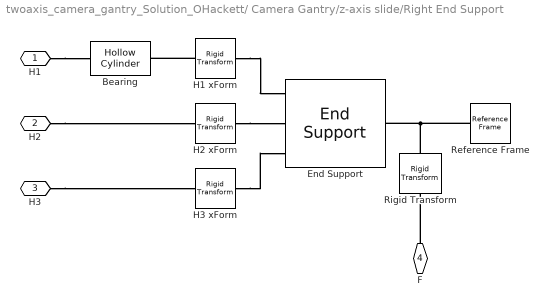
== system twoaxis_camera_gantry_Solution_OHackett/	Camera Gantry/z-axis slide/Right End Support ==
  Bearing : sm_linear_actuator_lib/Hollow Cylinder  StatePerturbationForJacobian=1.0e-05  R=R1+T  T=T  L=D  rho=rho  color=bColor
      settings: SourceProductBaseCode=MS
  End Support : sm_linear_actuator_lib/End Support  StatePerturbationForJacobian=1.0e-05  H=H  W=W  D=D  R1=R1+T  R2=R2  hole1_offset=hole1_offset  hole2_offset=hole2_offset  hole3_offset=hole3_offset  rho=rho  color=sColor
      settings: SourceProductBaseCode=MS
  H1 xForm : sm_lib/Frames and Transforms/Rigid Transform  StatePerturbationForJacobian=1.0e-05  TranslationMethod=None  TranslationStandardOffset=0  TranslationLengthUnit=m  TranslationStandardAxis=+Z  TranslationCartesianOffset=[0 0 0]  TranslationROffset=0  TranslationROffsetUnits=m  TranslationZOffset=0  TranslationZOffsetUnits=m  TranslationThetaOffset=0  TranslationThetaOffsetUnits=deg  RotationMethod=AlignedAxes  RotationAngleUnits=deg  RotationStandardAxis=+Z  RotationAngle=0.0  RotationArbitraryAxis=[0 0 1]  FollAlignAxisA=+Z  BaseAlignAxisA=-Z  FollAlignAxisB=+Y  BaseAlignAxisB=+Y  RotationSequenceAxes=FollowerAxes  RotationSequence=XYX  RotationSequenceAngles=[0 0 0]  RotationSequenceAnglesUnits=deg  RotationMatrix=[1 0 0; 0 1 0; 0 0 1]
  H2 xForm : sm_lib/Frames and Transforms/Rigid Transform  StatePerturbationForJacobian=1.0e-05  TranslationMethod=StandardAxis  TranslationStandardOffset=D/2  TranslationLengthUnit=mm  TranslationStandardAxis=+Z  TranslationCartesianOffset=[0 0 0]  TranslationROffset=0  TranslationROffsetUnits=m  TranslationZOffset=0  TranslationZOffsetUnits=m  TranslationThetaOffset=0  TranslationThetaOffsetUnits=deg  RotationMethod=AlignedAxes  RotationAngleUnits=deg  RotationStandardAxis=+Z  RotationAngle=0.0  RotationArbitraryAxis=[0 0 1]  FollAlignAxisA=+Z  BaseAlignAxisA=-Z  FollAlignAxisB=+Y  BaseAlignAxisB=+Y  RotationSequenceAxes=FollowerAxes  RotationSequence=XYX  RotationSequenceAngles=[0 0 0]  RotationSequenceAnglesUnits=deg  RotationMatrix=[1 0 0; 0 1 0; 0 0 1]
  H3 xForm : sm_lib/Frames and Transforms/Rigid Transform  StatePerturbationForJacobian=1.0e-05  TranslationMethod=StandardAxis  TranslationStandardOffset=D/2  TranslationLengthUnit=mm  TranslationStandardAxis=+Z  TranslationCartesianOffset=[0 0 0]  TranslationROffset=0  TranslationROffsetUnits=m  TranslationZOffset=0  TranslationZOffsetUnits=m  TranslationThetaOffset=0  TranslationThetaOffsetUnits=deg  RotationMethod=AlignedAxes  RotationAngleUnits=deg  RotationStandardAxis=+Z  RotationAngle=0.0  RotationArbitraryAxis=[0 0 1]  FollAlignAxisA=+Z  BaseAlignAxisA=-Z  FollAlignAxisB=+Y  BaseAlignAxisB=+Y  RotationSequenceAxes=FollowerAxes  RotationSequence=XYX  RotationSequenceAngles=[0 0 0]  RotationSequenceAnglesUnits=deg  RotationMatrix=[1 0 0; 0 1 0; 0 0 1]
  Reference Frame : sm_lib/Frames and Transforms/Reference Frame  StatePerturbationForJacobian=1.0e-05
  Rigid Transform : sm_lib/Frames and Transforms/Rigid Transform  TranslationMethod=StandardAxis  TranslationStandardOffset=D  TranslationLengthUnit=mm  TranslationStandardAxis=+Z  TranslationCartesianOffset=[0 0 0]  TranslationROffset=0  TranslationROffsetUnits=m  TranslationZOffset=0  TranslationZOffsetUnits=m  TranslationThetaOffset=0  TranslationThetaOffsetUnits=deg  RotationMethod=None  RotationAngleUnits=deg  RotationStandardAxis=+Z  RotationAngle=0.0  RotationArbitraryAxis=[0 0 1]  FollAlignAxisA=+X  BaseAlignAxisA=+Y  FollAlignAxisB=+Y  BaseAlignAxisB=+Z  RotationSequenceAxes=FollowerAxes  RotationSequence=XYX  RotationSequenceAngles=[0 0 0]  RotationSequenceAnglesUnits=deg  RotationMatrix=[1 0 0; 0 1 0; 0 0 1]
  H1 : PMIOPort  StatePerturbationForJacobian=1.0e-05  Side=Left
  H2 : PMIOPort  StatePerturbationForJacobian=1.0e-05  Port=2  Side=Left
  H3 : PMIOPort  StatePerturbationForJacobian=1.0e-05  Port=3  Side=Left
  F : PMIOPort  Port=4  Side=Right
  connections:
  Reference Frame/RConn1 -- End Support/LConn1 -- Rigid Transform/LConn1
  H3/RConn1 -- H3 xForm/RConn1
  H2/RConn1 -- H2 xForm/RConn1
  H1/RConn1 -- Bearing/LConn1
  H1 xForm/RConn1 -- Bearing/RConn1
  H2 xForm/LConn1 -- End Support/RConn2
  H3 xForm/LConn1 -- End Support/RConn3
  H1 xForm/LConn1 -- End Support/RConn1
  F/RConn1 -- Rigid Transform/RConn1

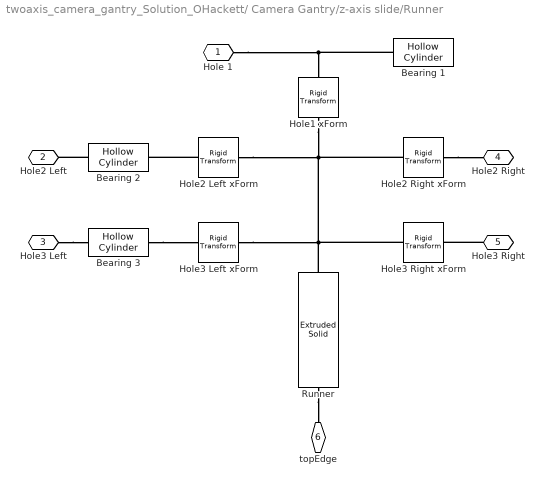
== system twoaxis_camera_gantry_Solution_OHackett/	Camera Gantry/z-axis slide/Runner ==
  Bearing 1 : sm_linear_actuator_lib/Hollow Cylinder  StatePerturbationForJacobian=1.0e-05  R=R1+T  T=T  L=D  rho=rho  color=bColor
      settings: SourceProductBaseCode=MS
  Bearing 2 : sm_linear_actuator_lib/Hollow Cylinder  StatePerturbationForJacobian=1.0e-05  R=R2+T  T=T  L=D  rho=rho  color=bColor
      settings: SourceProductBaseCode=MS
  Bearing 3 : sm_linear_actuator_lib/Hollow Cylinder  StatePerturbationForJacobian=1.0e-05  R=R2+T  T=T  L=D  rho=rho  color=bColor
      settings: SourceProductBaseCode=MS
  Hole1 xForm : sm_lib/Frames and Transforms/Rigid Transform  StatePerturbationForJacobian=1.0e-05  TranslationMethod=Cartesian  TranslationStandardOffset=0  TranslationLengthUnit=mm  TranslationStandardAxis=+Z  TranslationCartesianOffset=[hole1_offset 0]  TranslationROffset=0  TranslationROffsetUnits=m  TranslationZOffset=0  TranslationZOffsetUnits=m  TranslationThetaOffset=0  TranslationThetaOffsetUnits=deg  RotationMethod=None  RotationAngleUnits=deg  RotationStandardAxis=+Z  RotationAngle=0.0  RotationArbitraryAxis=[0 0 1]  FollAlignAxisA=+X  BaseAlignAxisA=+Y  FollAlignAxisB=+Y  BaseAlignAxisB=+Z  RotationSequenceAxes=FollowerAxes  RotationSequence=XYX  RotationSequenceAngles=[0 0 0]  RotationSequenceAnglesUnits=deg  RotationMatrix=[1 0 0; 0 1 0; 0 0 1]
  Hole2 Left xForm : sm_lib/Frames and Transforms/Rigid Transform  StatePerturbationForJacobian=1.0e-05  TranslationMethod=Cartesian  TranslationStandardOffset=0  TranslationLengthUnit=mm  TranslationStandardAxis=+Z  TranslationCartesianOffset=[hole2_offset 0]  TranslationROffset=0  TranslationROffsetUnits=m  TranslationZOffset=0  TranslationZOffsetUnits=m  TranslationThetaOffset=0  TranslationThetaOffsetUnits=deg  RotationMethod=None  RotationAngleUnits=deg  RotationStandardAxis=+Z  RotationAngle=0.0  RotationArbitraryAxis=[0 0 1]  FollAlignAxisA=+X  BaseAlignAxisA=+Y  FollAlignAxisB=+Y  BaseAlignAxisB=+Z  RotationSequenceAxes=FollowerAxes  RotationSequence=XYX  RotationSequenceAngles=[0 0 0]  RotationSequenceAnglesUnits=deg  RotationMatrix=[1 0 0; 0 1 0; 0 0 1]
  Hole2 Right xForm : sm_lib/Frames and Transforms/Rigid Transform  StatePerturbationForJacobian=1.0e-05  TranslationMethod=Cartesian  TranslationStandardOffset=0  TranslationLengthUnit=mm  TranslationStandardAxis=+Z  TranslationCartesianOffset=[hole2_offset D/2]  TranslationROffset=0  TranslationROffsetUnits=m  TranslationZOffset=0  TranslationZOffsetUnits=m  TranslationThetaOffset=0  TranslationThetaOffsetUnits=deg  RotationMethod=AlignedAxes  RotationAngleUnits=deg  RotationStandardAxis=+Z  RotationAngle=0.0  RotationArbitraryAxis=[0 0 1]  FollAlignAxisA=+Z  BaseAlignAxisA=-Z  FollAlignAxisB=+Y  BaseAlignAxisB=+Y  RotationSequenceAxes=FollowerAxes  RotationSequence=XYX  RotationSequenceAngles=[0 0 0]  RotationSequenceAnglesUnits=deg  RotationMatrix=[1 0 0; 0 1 0; 0 0 1]
  Hole3 Left xForm : sm_lib/Frames and Transforms/Rigid Transform  StatePerturbationForJacobian=1.0e-05  TranslationMethod=Cartesian  TranslationStandardOffset=0  TranslationLengthUnit=mm  TranslationStandardAxis=+Z  TranslationCartesianOffset=[hole3_offset 0]  TranslationROffset=0  TranslationROffsetUnits=m  TranslationZOffset=0  TranslationZOffsetUnits=m  TranslationThetaOffset=0  TranslationThetaOffsetUnits=deg  RotationMethod=None  RotationAngleUnits=deg  RotationStandardAxis=+Z  RotationAngle=0.0  RotationArbitraryAxis=[0 0 1]  FollAlignAxisA=+X  BaseAlignAxisA=+Y  FollAlignAxisB=+Y  BaseAlignAxisB=+Z  RotationSequenceAxes=FollowerAxes  RotationSequence=XYX  RotationSequenceAngles=[0 0 0]  RotationSequenceAnglesUnits=deg  RotationMatrix=[1 0 0; 0 1 0; 0 0 1]
  Hole3 Right xForm : sm_lib/Frames and Transforms/Rigid Transform  StatePerturbationForJacobian=1.0e-05  TranslationMethod=Cartesian  TranslationStandardOffset=0  TranslationLengthUnit=mm  TranslationStandardAxis=+Z  TranslationCartesianOffset=[hole3_offset D/2]  TranslationROffset=0  TranslationROffsetUnits=m  TranslationZOffset=0  TranslationZOffsetUnits=m  TranslationThetaOffset=0  TranslationThetaOffsetUnits=deg  RotationMethod=AlignedAxes  RotationAngleUnits=deg  RotationStandardAxis=+Z  RotationAngle=0.0  RotationArbitraryAxis=[0 0 1]  FollAlignAxisA=+Z  BaseAlignAxisA=-Z  FollAlignAxisB=+Y  BaseAlignAxisB=+Y  RotationSequenceAxes=FollowerAxes  RotationSequence=XYX  RotationSequenceAngles=[0 0 0]  RotationSequenceAnglesUnits=deg  RotationMatrix=[1 0 0; 0 1 0; 0 0 1]
  Runner : sm_lib/Body Elements/Extruded Solid  StatePerturbationForJacobian=1.0e-05  GraphicAmbientColor=[0.15 0.15 0.15 1.0]  BasedOnType=Density  CenterOfMass=[0 0 0]  CenterOfMassUnits=m  GraphicDiffuseColor=rColor  ExportConvexHullGeometry=off  ExtrusionCrossSection=extrusion_points  ExtrusionCrossSectionUnits=mm  Density=rho  DensityUnits=kg/(m^3)  DoExposeReferenceFrame=on  GraphicEmissiveColor=[0.0 0.0 0.0 1.0]  ExportEntireGeometry=off  ExtrusionLength=D  ExtrusionLengthUnits=mm  ExtrusionType=General  SerializedFrames=<Frames><Frame><Id>Frame1</Id><Value><Name>topEdge</Name><Origin><Source>GeometricFeature</Source><FeatureName>side curve 46</FeatureName></Origin><PrimaryAxis><DefinedDirection>+Z</DefinedDirection><Source>ReferenceFrame</Source><SourceDirection>+Z</SourceDirection><FeatureName></FeatureName></PrimaryAxis><SecondaryAxis><DefinedDirection>+X</DefinedDirection><Source>ReferenceFrame</Source><SourceDirection>+X</SourceDirection><FeatureName></FeatureName></SecondaryAxis></Value></Frame></Frames>  MarkerShape=Sphere  MarkerSize=10  GraphicType=FromGeometry  InertiaType=CalculateFromGeometry  Mass=1  MassUnits=kg  MomentsOfInertia=[1 1 1]  MomentsOfInertiaUnits=kg*m^2  PolygonNumSides=3  GraphicOpacity=0.9  PolygonOuterRadius=1  PolygonOuterRadiusUnits=m  ProductsOfInertia=[0 0 0]  ProductsOfInertiaUnits=kg*m^2  GraphicShininess=75  GraphicSpecularColor=[0.5 0.5 0.5 1.0]  GraphicVisPropType=SimpleVisualProperties
  Hole 1 : PMIOPort  StatePerturbationForJacobian=1.0e-05  Side=Left
  Hole2 Left : PMIOPort  StatePerturbationForJacobian=1.0e-05  Port=2  Side=Left
  Hole3 Left : PMIOPort  StatePerturbationForJacobian=1.0e-05  Port=3  Side=Left
  Hole2 Right : PMIOPort  StatePerturbationForJacobian=1.0e-05  Port=4  Side=Right
  Hole3 Right : PMIOPort  StatePerturbationForJacobian=1.0e-05  Port=5  Side=Right
  topEdge : PMIOPort  Port=6  Side=Right
  connections:
  Runner/LConn1 -- topEdge/RConn1
  Runner/RConn1 -- Hole2 Right xForm/LConn1 -- Hole2 Left xForm/LConn1 -- Hole1 xForm/LConn1 -- Hole3 Right xForm/LConn1 -- Hole3 Left xForm/LConn1
  Hole 1/RConn1 -- Hole1 xForm/RConn1 -- Bearing 1/RConn1
  Bearing 2/LConn1 -- Hole2 Left/RConn1
  Hole3 Right/RConn1 -- Hole3 Right xForm/RConn1
  Hole3 Left/RConn1 -- Bearing 3/LConn1
  Hole2 Right xForm/RConn1 -- Hole2 Right/RConn1
  Bearing 3/RConn1 -- Hole3 Left xForm/RConn1
  Hole2 Left xForm/RConn1 -- Bearing 2/RConn1
